simulink model "Control_model_10DOF_fin"  (R2016b)
(part 17 of 18)

JLcom(2,6)=(2*a2*mshank*cos(theta3 + theta4 - theta5 + theta6 + theta7 + theta8) - 2*lshank*mshank*cos(theta6 - theta3 - theta2 + theta7 + theta8) + 2*a2*mshank*cos(theta3 - theta4 + theta5 + theta6 + theta7 + theta8) + 2*a2*mthigh*cos(theta3 + theta4 - theta5 + theta6 + theta7 + theta8) + 2*a2*mthigh*cos(theta3 - theta4 + theta5 + theta6 + theta7 + theta8) - lthigh*mthigh*cos(theta3 + theta4 - theta5 + theta6 + theta7 + theta8) - lthigh*mthigh*cos(theta3 - theta4 + theta5 + theta6 + theta7 + theta8) + 4*a2*mshank*cos(theta6 - theta3 + theta7 + theta8) + 4*a2*mthigh*cos(theta6 - theta3 + theta7 + theta8) - 2*lthigh*mthigh*cos(theta6 - theta3 + theta7 + theta8) - 4*a4*mshank*sin(theta6 - theta5 + theta7 + theta8) - 4*a4*mthigh*sin(theta6 - theta5 + theta7 + theta8) - 4*a4*mtrunk*sin(theta6 - theta5 + theta7 + theta8) - 4*a1*mshank*cos(theta2 + theta3 + theta6 + theta7 + theta8) - 4*mtrunk*ypelvis*cos(theta6 - theta5 + theta7 + theta8) + 2*a1*mshank*cos(theta4 - theta3 - theta2 - theta5 + theta6 + theta7 + theta8) + 2*a1*mshank*cos(theta5 - theta3 - theta4 - theta2 + theta6 + theta7 + theta8) + 2*lshank*mshank*cos(theta2 + theta3 + theta6 + theta7 + theta8) + 4*mtrunk*xpelvis*sin(theta6 - theta5 + theta7 + theta8) - lshank*mshank*cos(theta4 - theta3 - theta2 - theta5 + theta6 + theta7 + theta8) - lshank*mshank*cos(theta5 - theta3 - theta4 - theta2 + theta6 + theta7 + theta8) + 2*a2*mshank*cos(theta4 - theta3 - theta5 + theta6 + theta7 + theta8) + 2*a2*mshank*cos(theta5 - theta4 - theta3 + theta6 + theta7 + theta8) + 2*a2*mthigh*cos(theta4 - theta3 - theta5 + theta6 + theta7 + theta8) + 2*a2*mthigh*cos(theta5 - theta4 - theta3 + theta6 + theta7 + theta8) - lthigh*mthigh*cos(theta4 - theta3 - theta5 + theta6 + theta7 + theta8) - lthigh*mthigh*cos(theta5 - theta4 - theta3 + theta6 + theta7 + theta8) - 8*mtrunk*zpelvis*sin(theta6 + theta7 + theta8) + 2*a1*mshank*cos(theta2 + theta3 + theta4 - theta5 + theta6 + theta7 + theta8) + 2*a1*mshank*cos(theta2 + theta3 - theta4 + theta5 + theta6 + theta7 + theta8) - lshank*mshank*cos(theta2 + theta3 + theta4 - theta5 + theta6 + theta7 + theta8) - lshank*mshank*cos(theta2 + theta3 - theta4 + theta5 + theta6 + theta7 + theta8) + 4*d3*mshank*sin(theta4 - theta5 + theta6 + theta7 + theta8) - 4*d3*mshank*sin(theta5 - theta4 + theta6 + theta7 + theta8) + 4*d3*mthigh*sin(theta4 - theta5 + theta6 + theta7 + theta8) - 4*d3*mthigh*sin(theta5 - theta4 + theta6 + theta7 + theta8) - 4*a2*mshank*cos(theta3 + theta6 + theta7 + theta8) - 4*a2*mthigh*cos(theta3 + theta6 + theta7 + theta8) + 2*lthigh*mthigh*cos(theta3 + theta6 + theta7 + theta8) + 4*a4*mshank*sin(theta5 + theta6 + theta7 + theta8) + 4*a4*mthigh*sin(theta5 + theta6 + theta7 + theta8) + 4*a4*mtrunk*sin(theta5 + theta6 + theta7 + theta8) - 4*mtrunk*ypelvis*cos(theta5 + theta6 + theta7 + theta8) - 4*mtrunk*xpelvis*sin(theta5 + theta6 + theta7 + theta8) + 4*a1*mshank*cos(theta6 - theta3 - theta2 + theta7 + theta8))/(8*(2*mshank + 2*mthigh + mtrunk));
JLcom(2,7)=(2*a2*mshank*cos(theta3 + theta4 - theta5 + theta6 + theta7 + theta8) - 2*lshank*mshank*cos(theta6 - theta3 - theta2 + theta7 + theta8) + 2*a2*mshank*cos(theta3 - theta4 + theta5 + theta6 + theta7 + theta8) + 2*a2*mthigh*cos(theta3 + theta4 - theta5 + theta6 + theta7 + theta8) + 2*a2*mthigh*cos(theta3 - theta4 + theta5 + theta6 + theta7 + theta8) - lthigh*mthigh*cos(theta3 + theta4 - theta5 + theta6 + theta7 + theta8) - lthigh*mthigh*cos(theta3 - theta4 + theta5 + theta6 + theta7 + theta8) + 4*a2*mshank*cos(theta6 - theta3 + theta7 + theta8) + 4*a2*mthigh*cos(theta6 - theta3 + theta7 + theta8) - 2*lthigh*mthigh*cos(theta6 - theta3 + theta7 + theta8) - 4*a4*mshank*sin(theta6 - theta5 + theta7 + theta8) - 4*a4*mthigh*sin(theta6 - theta5 + theta7 + theta8) - 4*a4*mtrunk*sin(theta6 - theta5 + theta7 + theta8) - 4*a1*mshank*cos(theta2 + theta3 + theta6 + theta7 + theta8) - 4*mtrunk*ypelvis*cos(theta6 - theta5 + theta7 + theta8) + 2*a1*mshank*cos(theta4 - theta3 - theta2 - theta5 + theta6 + theta7 + theta8) + 2*a1*mshank*cos(theta5 - theta3 - theta4 - theta2 + theta6 + theta7 + theta8) + 2*lshank*mshank*cos(theta2 + theta3 + theta6 + theta7 + theta8) + 4*mtrunk*xpelvis*sin(theta6 - theta5 + theta7 + theta8) - lshank*mshank*cos(theta4 - theta3 - theta2 - theta5 + theta6 + theta7 + theta8) - lshank*mshank*cos(theta5 - theta3 - theta4 - theta2 + theta6 + theta7 + theta8) + 2*a2*mshank*cos(theta4 - theta3 - theta5 + theta6 + theta7 + theta8) + 2*a2*mshank*cos(theta5 - theta4 - theta3 + theta6 + theta7 + theta8) + 2*a2*mthigh*cos(theta4 - theta3 - theta5 + theta6 + theta7 + theta8) + 2*a2*mthigh*cos(theta5 - theta4 - theta3 + theta6 + theta7 + theta8) - lthigh*mthigh*cos(theta4 - theta3 - theta5 + theta6 + theta7 + theta8) - lthigh*mthigh*cos(theta5 - theta4 - theta3 + theta6 + theta7 + theta8) - 8*mtrunk*zpelvis*sin(theta6 + theta7 + theta8) + 2*a1*mshank*cos(theta2 + theta3 + theta4 - theta5 + theta6 + theta7 + theta8) + 2*a1*mshank*cos(theta2 + theta3 - theta4 + theta5 + theta6 + theta7 + theta8) - lshank*mshank*cos(theta2 + theta3 + theta4 - theta5 + theta6 + theta7 + theta8) - lshank*mshank*cos(theta2 + theta3 - theta4 + theta5 + theta6 + theta7 + theta8) + 4*d3*mshank*sin(theta4 - theta5 + theta6 + theta7 + theta8) - 4*d3*mshank*sin(theta5 - theta4 + theta6 + theta7 + theta8) + 4*d3*mthigh*sin(theta4 - theta5 + theta6 + theta7 + theta8) - 4*d3*mthigh*sin(theta5 - theta4 + theta6 + theta7 + theta8) - 4*a2*mshank*cos(theta3 + theta6 + theta7 + theta8) - 4*a2*mthigh*cos(theta3 + theta6 + theta7 + theta8) + 2*lthigh*mthigh*cos(theta3 + theta6 + theta7 + theta8) + 4*a4*mshank*sin(theta5 + theta6 + theta7 + theta8) + 4*a4*mthigh*sin(theta5 + theta6 + theta7 + theta8) + 4*a4*mtrunk*sin(theta5 + theta6 + theta7 + theta8) + 8*a6*mshank*cos(theta7 + theta8) + 16*a6*mthigh*cos(theta7 + theta8) + 8*a6*mtrunk*cos(theta7 + theta8) - 4*mtrunk*ypelvis*cos(theta5 + theta6 + theta7 + theta8) + 4*lthigh*mthigh*cos(theta7 + theta8) - 4*mtrunk*xpelvis*sin(theta5 + theta6 + theta7 + theta8) + 4*a1*mshank*cos(theta6 - theta3 - theta2 + theta7 + theta8))/(8*(2*mshank + 2*mthigh + mtrunk));
JLcom(2,8)=(16*a7*mshank*cos(theta8) - 2*lshank*mshank*cos(theta6 - theta3 - theta2 + theta7 + theta8) + 16*a7*mthigh*cos(theta8) + 8*a7*mtrunk*cos(theta8) + 2*a2*mshank*cos(theta3 + theta4 - theta5 + theta6 + theta7 + theta8) + 2*a2*mshank*cos(theta3 - theta4 + theta5 + theta6 + theta7 + theta8) + 2*a2*mthigh*cos(theta3 + theta4 - theta5 + theta6 + theta7 + theta8) + 2*a2*mthigh*cos(theta3 - theta4 + theta5 + theta6 + theta7 + theta8) + 4*lshank*mshank*cos(theta8) - lthigh*mthigh*cos(theta3 + theta4 - theta5 + theta6 + theta7 + theta8) - lthigh*mthigh*cos(theta3 - theta4 + theta5 + theta6 + theta7 + theta8) + 4*a2*mshank*cos(theta6 - theta3 + theta7 + theta8) + 4*a2*mthigh*cos(theta6 - theta3 + theta7 + theta8) - 2*lthigh*mthigh*cos(theta6 - theta3 + theta7 + theta8) - 4*a4*mshank*sin(theta6 - theta5 + theta7 + theta8) - 4*a4*mthigh*sin(theta6 - theta5 + theta7 + theta8) - 4*a4*mtrunk*sin(theta6 - theta5 + theta7 + theta8) - 4*a1*mshank*cos(theta2 + theta3 + theta6 + theta7 + theta8) - 4*mtrunk*ypelvis*cos(theta6 - theta5 + theta7 + theta8) + 2*a1*mshank*cos(theta4 - theta3 - theta2 - theta5 + theta6 + theta7 + theta8) + 2*a1*mshank*cos(theta5 - theta3 - theta4 - theta2 + theta6 + theta7 + theta8) + 2*lshank*mshank*cos(theta2 + theta3 + theta6 + theta7 + theta8) + 4*mtrunk*xpelvis*sin(theta6 - theta5 + theta7 + theta8) - lshank*mshank*cos(theta4 - theta3 - theta2 - theta5 + theta6 + theta7 + theta8) - lshank*mshank*cos(theta5 - theta3 - theta4 - theta2 + theta6 + theta7 + theta8) + 2*a2*mshank*cos(theta4 - theta3 - theta5 + theta6 + theta7 + theta8) + 2*a2*mshank*cos(theta5 - theta4 - theta3 + theta6 + theta7 + theta8) + 2*a2*mthigh*cos(theta4 - theta3 - theta5 + theta6 + theta7 + theta8) + 2*a2*mthigh*cos(theta5 - theta4 - theta3 + theta6 + theta7 + theta8) - lthigh*mthigh*cos(theta4 - theta3 - theta5 + theta6 + theta7 + theta8) - lthigh*mthigh*cos(theta5 - theta4 - theta3 + theta6 + theta7 + theta8) - 8*mtrunk*zpelvis*sin(theta6 + theta7 + theta8) + 2*a1*mshank*cos(theta2 + theta3 + theta4 - theta5 + theta6 + theta7 + theta8) + 2*a1*mshank*cos(theta2 + theta3 - theta4 + theta5 + theta6 + theta7 + theta8) - lshank*mshank*cos(theta2 + theta3 + theta4 - theta5 + theta6 + theta7 + theta8) - lshank*mshank*cos(theta2 + theta3 - theta4 + theta5 + theta6 + theta7 + theta8) + 4*d3*mshank*sin(theta4 - theta5 + theta6 + theta7 + theta8) - 4*d3*mshank*sin(theta5 - theta4 + theta6 + theta7 + theta8) + 4*d3*mthigh*sin(theta4 - theta5 + theta6 + theta7 + theta8) - 4*d3*mthigh*sin(theta5 - theta4 + theta6 + theta7 + theta8) - 4*a2*mshank*cos(theta3 + theta6 + theta7 + theta8) - 4*a2*mthigh*cos(theta3 + theta6 + theta7 + theta8) + 2*lthigh*mthigh*cos(theta3 + theta6 + theta7 + theta8) + 4*a4*mshank*sin(theta5 + theta6 + theta7 + theta8) + 4*a4*mthigh*sin(theta5 + theta6 + theta7 + theta8) + 4*a4*mtrunk*sin(theta5 + theta6 + theta7 + theta8) + 8*a6*mshank*cos(theta7 + theta8) + 16*a6*mthigh*cos(theta7 + theta8) + 8*a6*mtrunk*cos(theta7 + theta8) - 4*mtrunk*ypelvis*cos(theta5 + theta6 + theta7 + theta8) + 4*lthigh*mthigh*cos(theta7 + theta8) - 4*mtrunk*xpelvis*sin(theta5 + theta6 + theta7 + theta8) + 4*a1*mshank*cos(theta6 - theta3 - theta2 + theta7 + theta8))/(8*(2*mshank + 2*mthigh + mtrunk));

JLcom(3,5)=(2*a4*mshank*cos(theta9)*sin(theta5) - 2*mtrunk*xpelvis*cos(theta9)*sin(theta5) + 2*a4*mthigh*cos(theta9)*sin(theta5) + 2*a4*mtrunk*cos(theta9)*sin(theta5) - 2*mtrunk*ypelvis*cos(theta5)*cos(theta9) - 2*d3*mshank*cos(theta4)*cos(theta9)*sin(theta5) + 2*d3*mshank*cos(theta5)*cos(theta9)*sin(theta4) - 2*d3*mthigh*cos(theta4)*cos(theta9)*sin(theta5) + 2*d3*mthigh*cos(theta5)*cos(theta9)*sin(theta4) + 2*a2*mshank*cos(theta3)*cos(theta4)*cos(theta5)*cos(theta9) + 2*a2*mthigh*cos(theta3)*cos(theta4)*cos(theta5)*cos(theta9) - lthigh*mthigh*cos(theta3)*cos(theta4)*cos(theta5)*cos(theta9) + 2*a2*mshank*cos(theta3)*cos(theta9)*sin(theta4)*sin(theta5) + 2*a2*mthigh*cos(theta3)*cos(theta9)*sin(theta4)*sin(theta5) - lthigh*mthigh*cos(theta3)*cos(theta9)*sin(theta4)*sin(theta5) + 2*a1*mshank*cos(theta2)*cos(theta3)*cos(theta4)*cos(theta5)*cos(theta9) - lshank*mshank*cos(theta2)*cos(theta3)*cos(theta4)*cos(theta5)*cos(theta9) + 2*a4*mshank*cos(theta5)*cos(theta6)*cos(theta7)*cos(theta8)*sin(theta9) + 2*a4*mthigh*cos(theta5)*cos(theta6)*cos(theta7)*cos(theta8)*sin(theta9) + 2*a4*mtrunk*cos(theta5)*cos(theta6)*cos(theta7)*cos(theta8)*sin(theta9) + 2*a1*mshank*cos(theta2)*cos(theta3)*cos(theta9)*sin(theta4)*sin(theta5) - 2*a1*mshank*cos(theta4)*cos(theta5)*cos(theta9)*sin(theta2)*sin(theta3) - 2*mtrunk*xpelvis*cos(theta5)*cos(theta6)*cos(theta7)*cos(theta8)*sin(theta9) - lshank*mshank*cos(theta2)*cos(theta3)*cos(theta9)*sin(theta4)*sin(theta5) + lshank*mshank*cos(theta4)*cos(theta5)*cos(theta9)*sin(theta2)*sin(theta3) - 2*a4*mshank*cos(theta5)*cos(theta6)*sin(theta7)*sin(theta8)*sin(theta9) - 2*a4*mshank*cos(theta5)*cos(theta7)*sin(theta6)*sin(theta8)*sin(theta9) - 2*a4*mshank*cos(theta5)*cos(theta8)*sin(theta6)*sin(theta7)*sin(theta9) - 2*a4*mthigh*cos(theta5)*cos(theta6)*sin(theta7)*sin(theta8)*sin(theta9) - 2*a4*mthigh*cos(theta5)*cos(theta7)*sin(theta6)*sin(theta8)*sin(theta9) - 2*a4*mthigh*cos(theta5)*cos(theta8)*sin(theta6)*sin(theta7)*sin(theta9) - 2*a4*mtrunk*cos(theta5)*cos(theta6)*sin(theta7)*sin(theta8)*sin(theta9) - 2*a4*mtrunk*cos(theta5)*cos(theta7)*sin(theta6)*sin(theta8)*sin(theta9) - 2*a4*mtrunk*cos(theta5)*cos(theta8)*sin(theta6)*sin(theta7)*sin(theta9) + 2*mtrunk*ypelvis*cos(theta6)*cos(theta7)*cos(theta8)*sin(theta5)*sin(theta9) - 2*a1*mshank*cos(theta9)*sin(theta2)*sin(theta3)*sin(theta4)*sin(theta5) + 2*mtrunk*xpelvis*cos(theta5)*cos(theta6)*sin(theta7)*sin(theta8)*sin(theta9) + 2*mtrunk*xpelvis*cos(theta5)*cos(theta7)*sin(theta6)*sin(theta8)*sin(theta9) + 2*mtrunk*xpelvis*cos(theta5)*cos(theta8)*sin(theta6)*sin(theta7)*sin(theta9) + lshank*mshank*cos(theta9)*sin(theta2)*sin(theta3)*sin(theta4)*sin(theta5) - 2*mtrunk*ypelvis*cos(theta6)*sin(theta5)*sin(theta7)*sin(theta8)*sin(theta9) - 2*mtrunk*ypelvis*cos(theta7)*sin(theta5)*sin(theta6)*sin(theta8)*sin(theta9) - 2*mtrunk*ypelvis*cos(theta8)*sin(theta5)*sin(theta6)*sin(theta7)*sin(theta9) - 2*d3*mshank*cos(theta4)*cos(theta5)*cos(theta6)*cos(theta7)*cos(theta8)*sin(theta9) - 2*d3*mthigh*cos(theta4)*cos(theta5)*cos(theta6)*cos(theta7)*cos(theta8)*sin(theta9) + 2*d3*mshank*cos(theta4)*cos(theta5)*cos(theta6)*sin(theta7)*sin(theta8)*sin(theta9) + 2*d3*mshank*cos(theta4)*cos(theta5)*cos(theta7)*sin(theta6)*sin(theta8)*sin(theta9) + 2*d3*mshank*cos(theta4)*cos(theta5)*cos(theta8)*sin(theta6)*sin(theta7)*sin(theta9) - 2*d3*mshank*cos(theta6)*cos(theta7)*cos(theta8)*sin(theta4)*sin(theta5)*sin(theta9) + 2*d3*mthigh*cos(theta4)*cos(theta5)*cos(theta6)*sin(theta7)*sin(theta8)*sin(theta9) + 2*d3*mthigh*cos(theta4)*cos(theta5)*cos(theta7)*sin(theta6)*sin(theta8)*sin(theta9) + 2*d3*mthigh*cos(theta4)*cos(theta5)*cos(theta8)*sin(theta6)*sin(theta7)*sin(theta9) - 2*d3*mthigh*cos(theta6)*cos(theta7)*cos(theta8)*sin(theta4)*sin(theta5)*sin(theta9) + 2*d3*mshank*cos(theta6)*sin(theta4)*sin(theta5)*sin(theta7)*sin(theta8)*sin(theta9) + 2*d3*mshank*cos(theta7)*sin(theta4)*sin(theta5)*sin(theta6)*sin(theta8)*sin(theta9) + 2*d3*mshank*cos(theta8)*sin(theta4)*sin(theta5)*sin(theta6)*sin(theta7)*sin(theta9) + 2*d3*mthigh*cos(theta6)*sin(theta4)*sin(theta5)*sin(theta7)*sin(theta8)*sin(theta9) + 2*d3*mthigh*cos(theta7)*sin(theta4)*sin(theta5)*sin(theta6)*sin(theta8)*sin(theta9) + 2*d3*mthigh*cos(theta8)*sin(theta4)*sin(theta5)*sin(theta6)*sin(theta7)*sin(theta9) - 2*a2*mshank*cos(theta3)*cos(theta4)*cos(theta6)*cos(theta7)*cos(theta8)*sin(theta5)*sin(theta9) + 2*a2*mshank*cos(theta3)*cos(theta5)*cos(theta6)*cos(theta7)*cos(theta8)*sin(theta4)*sin(theta9) - 2*a2*mthigh*cos(theta3)*cos(theta4)*cos(theta6)*cos(theta7)*cos(theta8)*sin(theta5)*sin(theta9) + 2*a2*mthigh*cos(theta3)*cos(theta5)*cos(theta6)*cos(theta7)*cos(theta8)*sin(theta4)*sin(theta9) + lthigh*mthigh*cos(theta3)*cos(theta4)*cos(theta6)*cos(theta7)*cos(theta8)*sin(theta5)*sin(theta9) - lthigh*mthigh*cos(theta3)*cos(theta5)*cos(theta6)*cos(theta7)*cos(theta8)*sin(theta4)*sin(theta9) + 2*a2*mshank*cos(theta3)*cos(theta4)*cos(theta6)*sin(theta5)*sin(theta7)*sin(theta8)*sin(theta9) + 2*a2*mshank*cos(theta3)*cos(theta4)*cos(theta7)*sin(theta5)*sin(theta6)*sin(theta8)*sin(theta9) + 2*a2*mshank*cos(theta3)*cos(theta4)*cos(theta8)*sin(theta5)*sin(theta6)*sin(theta7)*sin(theta9) - 2*a2*mshank*cos(theta3)*cos(theta5)*cos(theta6)*sin(theta4)*sin(theta7)*sin(theta8)*sin(theta9) - 2*a2*mshank*cos(theta3)*cos(theta5)*cos(theta7)*sin(theta4)*sin(theta6)*sin(theta8)*sin(theta9) - 2*a2*mshank*cos(theta3)*cos(theta5)*cos(theta8)*sin(theta4)*sin(theta6)*sin(theta7)*sin(theta9) + 2*a2*mthigh*cos(theta3)*cos(theta4)*cos(theta6)*sin(theta5)*sin(theta7)*sin(theta8)*sin(theta9) + 2*a2*mthigh*cos(theta3)*cos(theta4)*cos(theta7)*sin(theta5)*sin(theta6)*sin(theta8)*sin(theta9) + 2*a2*mthigh*cos(theta3)*cos(theta4)*cos(theta8)*sin(theta5)*sin(theta6)*sin(theta7)*sin(theta9) - 2*a2*mthigh*cos(theta3)*cos(theta5)*cos(theta6)*sin(theta4)*sin(theta7)*sin(theta8)*sin(theta9) - 2*a2*mthigh*cos(theta3)*cos(theta5)*cos(theta7)*sin(theta4)*sin(theta6)*sin(theta8)*sin(theta9) - 2*a2*mthigh*cos(theta3)*cos(theta5)*cos(theta8)*sin(theta4)*sin(theta6)*sin(theta7)*sin(theta9) - lthigh*mthigh*cos(theta3)*cos(theta4)*cos(theta6)*sin(theta5)*sin(theta7)*sin(theta8)*sin(theta9) - lthigh*mthigh*cos(theta3)*cos(theta4)*cos(theta7)*sin(theta5)*sin(theta6)*sin(theta8)*sin(theta9) - lthigh*mthigh*cos(theta3)*cos(theta4)*cos(theta8)*sin(theta5)*sin(theta6)*sin(theta7)*sin(theta9) + lthigh*mthigh*cos(theta3)*cos(theta5)*cos(theta6)*sin(theta4)*sin(theta7)*sin(theta8)*sin(theta9) + lthigh*mthigh*cos(theta3)*cos(theta5)*cos(theta7)*sin(theta4)*sin(theta6)*sin(theta8)*sin(theta9) + lthigh*mthigh*cos(theta3)*cos(theta5)*cos(theta8)*sin(theta4)*sin(theta6)*sin(theta7)*sin(theta9) - 2*a1*mshank*cos(theta2)*cos(theta3)*cos(theta4)*cos(theta6)*cos(theta7)*cos(theta8)*sin(theta5)*sin(theta9) + 2*a1*mshank*cos(theta2)*cos(theta3)*cos(theta5)*cos(theta6)*cos(theta7)*cos(theta8)*sin(theta4)*sin(theta9) + lshank*mshank*cos(theta2)*cos(theta3)*cos(theta4)*cos(theta6)*cos(theta7)*cos(theta8)*sin(theta5)*sin(theta9) - lshank*mshank*cos(theta2)*cos(theta3)*cos(theta5)*cos(theta6)*cos(theta7)*cos(theta8)*sin(theta4)*sin(theta9) + 2*a1*mshank*cos(theta2)*cos(theta3)*cos(theta4)*cos(theta6)*sin(theta5)*sin(theta7)*sin(theta8)*sin(theta9) + 2*a1*mshank*cos(theta2)*cos(theta3)*cos(theta4)*cos(theta7)*sin(theta5)*sin(theta6)*sin(theta8)*sin(theta9) + 2*a1*mshank*cos(theta2)*cos(theta3)*cos(theta4)*cos(theta8)*sin(theta5)*sin(theta6)*sin(theta7)*sin(theta9) - 2*a1*mshank*cos(theta2)*cos(theta3)*cos(theta5)*cos(theta6)*sin(theta4)*sin(theta7)*sin(theta8)*sin(theta9) - 2*a1*mshank*cos(theta2)*cos(theta3)*cos(theta5)*cos(theta7)*sin(theta4)*sin(theta6)*sin(theta8)*sin(theta9) - 2*a1*mshank*cos(theta2)*cos(theta3)*cos(theta5)*cos(theta8)*sin(theta4)*sin(theta6)*sin(theta7)*sin(theta9) + 2*a1*mshank*cos(theta4)*cos(theta6)*cos(theta7)*cos(theta8)*sin(theta2)*sin(theta3)*sin(theta5)*sin(theta9) - 2*a1*mshank*cos(theta5)*cos(theta6)*cos(theta7)*cos(theta8)*sin(theta2)*sin(theta3)*sin(theta4)*sin(theta9) - lshank*mshank*cos(theta2)*cos(theta3)*cos(theta4)*cos(theta6)*sin(theta5)*sin(theta7)*sin(theta8)*sin(theta9) - lshank*mshank*cos(theta2)*cos(theta3)*cos(theta4)*cos(theta7)*sin(theta5)*sin(theta6)*sin(theta8)*sin(theta9) - lshank*mshank*cos(theta2)*cos(theta3)*cos(theta4)*cos(theta8)*sin(theta5)*sin(theta6)*sin(theta7)*sin(theta9) + lshank*mshank*cos(theta2)*cos(theta3)*cos(theta5)*cos(theta6)*sin(theta4)*sin(theta7)*sin(theta8)*sin(theta9) + lshank*mshank*cos(theta2)*cos(theta3)*cos(theta5)*cos(theta7)*sin(theta4)*sin(theta6)*sin(theta8)*sin(theta9) + lshank*mshank*cos(theta2)*cos(theta3)*cos(theta5)*cos(theta8)*sin(theta4)*sin(theta6)*sin(theta7)*sin(theta9) - lshank*mshank*cos(theta4)*cos(theta6)*cos(theta7)*cos(theta8)*sin(theta2)*sin(theta3)*sin(theta5)*sin(theta9) + lshank*mshank*cos(theta5)*cos(theta6)*cos(theta7)*cos(theta8)*sin(theta2)*sin(theta3)*sin(theta4)*sin(theta9) - 2*a1*mshank*cos(theta4)*cos(theta6)*sin(theta2)*sin(theta3)*sin(theta5)*sin(theta7)*sin(theta8)*sin(theta9) - 2*a1*mshank*cos(theta4)*cos(theta7)*sin(theta2)*sin(theta3)*sin(theta5)*sin(theta6)*sin(theta8)*sin(theta9) - 2*a1*mshank*cos(theta4)*cos(theta8)*sin(theta2)*sin(theta3)*sin(theta5)*sin(theta6)*sin(theta7)*sin(theta9) + 2*a1*mshank*cos(theta5)*cos(theta6)*sin(theta2)*sin(theta3)*sin(theta4)*sin(theta7)*sin(theta8)*sin(theta9) + 2*a1*mshank*cos(theta5)*cos(theta7)*sin(theta2)*sin(theta3)*sin(theta4)*sin(theta6)*sin(theta8)*sin(theta9) + 2*a1*mshank*cos(theta5)*cos(theta8)*sin(theta2)*sin(theta3)*sin(theta4)*sin(theta6)*sin(theta7)*sin(theta9) + lshank*mshank*cos(theta4)*cos(theta6)*sin(theta2)*sin(theta3)*sin(theta5)*sin(theta7)*sin(theta8)*sin(theta9) + lshank*mshank*cos(theta4)*cos(theta7)*sin(theta2)*sin(theta3)*sin(theta5)*sin(theta6)*sin(theta8)*sin(theta9) + lshank*mshank*cos(theta4)*cos(theta8)*sin(theta2)*sin(theta3)*sin(theta5)*sin(theta6)*sin(theta7)*sin(theta9) - lshank*mshank*cos(theta5)*cos(theta6)*sin(theta2)*sin(theta3)*sin(theta4)*sin(theta7)*sin(theta8)*sin(theta9) - lshank*mshank*cos(theta5)*cos(theta7)*sin(theta2)*sin(theta3)*sin(theta4)*sin(theta6)*sin(theta8)*sin(theta9) - lshank*mshank*cos(theta5)*cos(theta8)*sin(theta2)*sin(theta3)*sin(theta4)*sin(theta6)*sin(theta7)*sin(theta9))/(4*mshank + 4*mthigh + 2*mtrunk);
JLcom(3,6)=-(2*mtrunk*zpelvis*cos(theta6)*cos(theta7)*cos(theta8)*sin(theta9) - 2*mtrunk*zpelvis*cos(theta6)*sin(theta7)*sin(theta8)*sin(theta9) - 2*mtrunk*zpelvis*cos(theta7)*sin(theta6)*sin(theta8)*sin(theta9) - 2*mtrunk*zpelvis*cos(theta8)*sin(theta6)*sin(theta7)*sin(theta9) - 2*a2*mshank*cos(theta6)*cos(theta7)*cos(theta8)*sin(theta3)*sin(theta9) - 2*a2*mthigh*cos(theta6)*cos(theta7)*cos(theta8)*sin(theta3)*sin(theta9) + lthigh*mthigh*cos(theta6)*cos(theta7)*cos(theta8)*sin(theta3)*sin(theta9) + 2*a4*mshank*cos(theta6)*cos(theta7)*sin(theta5)*sin(theta8)*sin(theta9) + 2*a4*mshank*cos(theta6)*cos(theta8)*sin(theta5)*sin(theta7)*sin(theta9) + 2*a4*mshank*cos(theta7)*cos(theta8)*sin(theta5)*sin(theta6)*sin(theta9) + 2*a4*mthigh*cos(theta6)*cos(theta7)*sin(theta5)*sin(theta8)*sin(theta9) + 2*a4*mthigh*cos(theta6)*cos(theta8)*sin(theta5)*sin(theta7)*sin(theta9) + 2*a4*mthigh*cos(theta7)*cos(theta8)*sin(theta5)*sin(theta6)*sin(theta9) + 2*a4*mtrunk*cos(theta6)*cos(theta7)*sin(theta5)*sin(theta8)*sin(theta9) + 2*a4*mtrunk*cos(theta6)*cos(theta8)*sin(theta5)*sin(theta7)*sin(theta9) + 2*a4*mtrunk*cos(theta7)*cos(theta8)*sin(theta5)*sin(theta6)*sin(theta9) - 2*mtrunk*ypelvis*cos(theta5)*cos(theta6)*cos(theta7)*sin(theta8)*sin(theta9) - 2*mtrunk*ypelvis*cos(theta5)*cos(theta6)*cos(theta8)*sin(theta7)*sin(theta9) - 2*mtrunk*ypelvis*cos(theta5)*cos(theta7)*cos(theta8)*sin(theta6)*sin(theta9) + 2*a2*mshank*cos(theta6)*sin(theta3)*sin(theta7)*sin(theta8)*sin(theta9) + 2*a2*mshank*cos(theta7)*sin(theta3)*sin(theta6)*sin(theta8)*sin(theta9) + 2*a2*mshank*cos(theta8)*sin(theta3)*sin(theta6)*sin(theta7)*sin(theta9) + 2*a2*mthigh*cos(theta6)*sin(theta3)*sin(theta7)*sin(theta8)*sin(theta9) + 2*a2*mthigh*cos(theta7)*sin(theta3)*sin(theta6)*sin(theta8)*sin(theta9) + 2*a2*mthigh*cos(theta8)*sin(theta3)*sin(theta6)*sin(theta7)*sin(theta9) - 2*mtrunk*xpelvis*cos(theta6)*cos(theta7)*sin(theta5)*sin(theta8)*sin(theta9) - 2*mtrunk*xpelvis*cos(theta6)*cos(theta8)*sin(theta5)*sin(theta7)*sin(theta9) - 2*mtrunk*xpelvis*cos(theta7)*cos(theta8)*sin(theta5)*sin(theta6)*sin(theta9) - lthigh*mthigh*cos(theta6)*sin(theta3)*sin(theta7)*sin(theta8)*sin(theta9) - lthigh*mthigh*cos(theta7)*sin(theta3)*sin(theta6)*sin(theta8)*sin(theta9) - lthigh*mthigh*cos(theta8)*sin(theta3)*sin(theta6)*sin(theta7)*sin(theta9) - 2*a4*mshank*sin(theta5)*sin(theta6)*sin(theta7)*sin(theta8)*sin(theta9) - 2*a4*mthigh*sin(theta5)*sin(theta6)*sin(theta7)*sin(theta8)*sin(theta9) - 2*a4*mtrunk*sin(theta5)*sin(theta6)*sin(theta7)*sin(theta8)*sin(theta9) + 2*mtrunk*ypelvis*cos(theta5)*sin(theta6)*sin(theta7)*sin(theta8)*sin(theta9) + 2*mtrunk*xpelvis*sin(theta5)*sin(theta6)*sin(theta7)*sin(theta8)*sin(theta9) - 2*a1*mshank*cos(theta2)*cos(theta6)*cos(theta7)*cos(theta8)*sin(theta3)*sin(theta9) - 2*a1*mshank*cos(theta3)*cos(theta6)*cos(theta7)*cos(theta8)*sin(theta2)*sin(theta9) + lshank*mshank*cos(theta2)*cos(theta6)*cos(theta7)*cos(theta8)*sin(theta3)*sin(theta9) + lshank*mshank*cos(theta3)*cos(theta6)*cos(theta7)*cos(theta8)*sin(theta2)*sin(theta9) - 2*d3*mshank*cos(theta4)*cos(theta6)*cos(theta7)*sin(theta5)*sin(theta8)*sin(theta9) - 2*d3*mshank*cos(theta4)*cos(theta6)*cos(theta8)*sin(theta5)*sin(theta7)*sin(theta9) - 2*d3*mshank*cos(theta4)*cos(theta7)*cos(theta8)*sin(theta5)*sin(theta6)*sin(theta9) + 2*d3*mshank*cos(theta5)*cos(theta6)*cos(theta7)*sin(theta4)*sin(theta8)*sin(theta9) + 2*d3*mshank*cos(theta5)*cos(theta6)*cos(theta8)*sin(theta4)*sin(theta7)*sin(theta9) + 2*d3*mshank*cos(theta5)*cos(theta7)*cos(theta8)*sin(theta4)*sin(theta6)*sin(theta9) - 2*d3*mthigh*cos(theta4)*cos(theta6)*cos(theta7)*sin(theta5)*sin(theta8)*sin(theta9) - 2*d3*mthigh*cos(theta4)*cos(theta6)*cos(theta8)*sin(theta5)*sin(theta7)*sin(theta9) - 2*d3*mthigh*cos(theta4)*cos(theta7)*cos(theta8)*sin(theta5)*sin(theta6)*sin(theta9) + 2*d3*mthigh*cos(theta5)*cos(theta6)*cos(theta7)*sin(theta4)*sin(theta8)*sin(theta9) + 2*d3*mthigh*cos(theta5)*cos(theta6)*cos(theta8)*sin(theta4)*sin(theta7)*sin(theta9) + 2*d3*mthigh*cos(theta5)*cos(theta7)*cos(theta8)*sin(theta4)*sin(theta6)*sin(theta9) + 2*a1*mshank*cos(theta2)*cos(theta6)*sin(theta3)*sin(theta7)*sin(theta8)*sin(theta9) + 2*a1*mshank*cos(theta2)*cos(theta7)*sin(theta3)*sin(theta6)*sin(theta8)*sin(theta9) + 2*a1*mshank*cos(theta2)*cos(theta8)*sin(theta3)*sin(theta6)*sin(theta7)*sin(theta9) + 2*a1*mshank*cos(theta3)*cos(theta6)*sin(theta2)*sin(theta7)*sin(theta8)*sin(theta9) + 2*a1*mshank*cos(theta3)*cos(theta7)*sin(theta2)*sin(theta6)*sin(theta8)*sin(theta9) + 2*a1*mshank*cos(theta3)*cos(theta8)*sin(theta2)*sin(theta6)*sin(theta7)*sin(theta9) - lshank*mshank*cos(theta2)*cos(theta6)*sin(theta3)*sin(theta7)*sin(theta8)*sin(theta9) - lshank*mshank*cos(theta2)*cos(theta7)*sin(theta3)*sin(theta6)*sin(theta8)*sin(theta9) - lshank*mshank*cos(theta2)*cos(theta8)*sin(theta3)*sin(theta6)*sin(theta7)*sin(theta9) - lshank*mshank*cos(theta3)*cos(theta6)*sin(theta2)*sin(theta7)*sin(theta8)*sin(theta9) - lshank*mshank*cos(theta3)*cos(theta7)*sin(theta2)*sin(theta6)*sin(theta8)*sin(theta9) - lshank*mshank*cos(theta3)*cos(theta8)*sin(theta2)*sin(theta6)*sin(theta7)*sin(theta9) + 2*d3*mshank*cos(theta4)*sin(theta5)*sin(theta6)*sin(theta7)*sin(theta8)*sin(theta9) - 2*d3*mshank*cos(theta5)*sin(theta4)*sin(theta6)*sin(theta7)*sin(theta8)*sin(theta9) + 2*d3*mthigh*cos(theta4)*sin(theta5)*sin(theta6)*sin(theta7)*sin(theta8)*sin(theta9) - 2*d3*mthigh*cos(theta5)*sin(theta4)*sin(theta6)*sin(theta7)*sin(theta8)*sin(theta9) + 2*a2*mshank*cos(theta3)*cos(theta4)*cos(theta5)*cos(theta6)*cos(theta7)*sin(theta8)*sin(theta9) + 2*a2*mshank*cos(theta3)*cos(theta4)*cos(theta5)*cos(theta6)*cos(theta8)*sin(theta7)*sin(theta9) + 2*a2*mshank*cos(theta3)*cos(theta4)*cos(theta5)*cos(theta7)*cos(theta8)*sin(theta6)*sin(theta9) + 2*a2*mthigh*cos(theta3)*cos(theta4)*cos(theta5)*cos(theta6)*cos(theta7)*sin(theta8)*sin(theta9) + 2*a2*mthigh*cos(theta3)*cos(theta4)*cos(theta5)*cos(theta6)*cos(theta8)*sin(theta7)*sin(theta9) + 2*a2*mthigh*cos(theta3)*cos(theta4)*cos(theta5)*cos(theta7)*cos(theta8)*sin(theta6)*sin(theta9) - lthigh*mthigh*cos(theta3)*cos(theta4)*cos(theta5)*cos(theta6)*cos(theta7)*sin(theta8)*sin(theta9) - lthigh*mthigh*cos(theta3)*cos(theta4)*cos(theta5)*cos(theta6)*cos(theta8)*sin(theta7)*sin(theta9) - lthigh*mthigh*cos(theta3)*cos(theta4)*cos(theta5)*cos(theta7)*cos(theta8)*sin(theta6)*sin(theta9) - 2*a2*mshank*cos(theta3)*cos(theta4)*cos(theta5)*sin(theta6)*sin(theta7)*sin(theta8)*sin(theta9) + 2*a2*mshank*cos(theta3)*cos(theta6)*cos(theta7)*sin(theta4)*sin(theta5)*sin(theta8)*sin(theta9) + 2*a2*mshank*cos(theta3)*cos(theta6)*cos(theta8)*sin(theta4)*sin(theta5)*sin(theta7)*sin(theta9) + 2*a2*mshank*cos(theta3)*cos(theta7)*cos(theta8)*sin(theta4)*sin(theta5)*sin(theta6)*sin(theta9) - 2*a2*mthigh*cos(theta3)*cos(theta4)*cos(theta5)*sin(theta6)*sin(theta7)*sin(theta8)*sin(theta9) + 2*a2*mthigh*cos(theta3)*cos(theta6)*cos(theta7)*sin(theta4)*sin(theta5)*sin(theta8)*sin(theta9) + 2*a2*mthigh*cos(theta3)*cos(theta6)*cos(theta8)*sin(theta4)*sin(theta5)*sin(theta7)*sin(theta9) + 2*a2*mthigh*cos(theta3)*cos(theta7)*cos(theta8)*sin(theta4)*sin(theta5)*sin(theta6)*sin(theta9) + lthigh*mthigh*cos(theta3)*cos(theta4)*cos(theta5)*sin(theta6)*sin(theta7)*sin(theta8)*sin(theta9) - lthigh*mthigh*cos(theta3)*cos(theta6)*cos(theta7)*sin(theta4)*sin(theta5)*sin(theta8)*sin(theta9) - lthigh*mthigh*cos(theta3)*cos(theta6)*cos(theta8)*sin(theta4)*sin(theta5)*sin(theta7)*sin(theta9) - lthigh*mthigh*cos(theta3)*cos(theta7)*cos(theta8)*sin(theta4)*sin(theta5)*sin(theta6)*sin(theta9) - 2*a2*mshank*cos(theta3)*sin(theta4)*sin(theta5)*sin(theta6)*sin(theta7)*sin(theta8)*sin(theta9) - 2*a2*mthigh*cos(theta3)*sin(theta4)*sin(theta5)*sin(theta6)*sin(theta7)*sin(theta8)*sin(theta9) + lthigh*mthigh*cos(theta3)*sin(theta4)*sin(theta5)*sin(theta6)*sin(theta7)*sin(theta8)*sin(theta9) + 2*a1*mshank*cos(theta2)*cos(theta3)*cos(theta4)*cos(theta5)*cos(theta6)*cos(theta7)*sin(theta8)*sin(theta9) + 2*a1*mshank*cos(theta2)*cos(theta3)*cos(theta4)*cos(theta5)*cos(theta6)*cos(theta8)*sin(theta7)*sin(theta9) + 2*a1*mshank*cos(theta2)*cos(theta3)*cos(theta4)*cos(theta5)*cos(theta7)*cos(theta8)*sin(theta6)*sin(theta9) - lshank*mshank*cos(theta2)*cos(theta3)*cos(theta4)*cos(theta5)*cos(theta6)*cos(theta7)*sin(theta8)*sin(theta9) - lshank*mshank*cos(theta2)*cos(theta3)*cos(theta4)*cos(theta5)*cos(theta6)*cos(theta8)*sin(theta7)*sin(theta9) - lshank*mshank*cos(theta2)*cos(theta3)*cos(theta4)*cos(theta5)*cos(theta7)*cos(theta8)*sin(theta6)*sin(theta9) - 2*a1*mshank*cos(theta2)*cos(theta3)*cos(theta4)*cos(theta5)*sin(theta6)*sin(theta7)*sin(theta8)*sin(theta9) + 2*a1*mshank*cos(theta2)*cos(theta3)*cos(theta6)*cos(theta7)*sin(theta4)*sin(theta5)*sin(theta8)*sin(theta9) + 2*a1*mshank*cos(theta2)*cos(theta3)*cos(theta6)*cos(theta8)*sin(theta4)*sin(theta5)*sin(theta7)*sin(theta9) + 2*a1*mshank*cos(theta2)*cos(theta3)*cos(theta7)*cos(theta8)*sin(theta4)*sin(theta5)*sin(theta6)*sin(theta9) - 2*a1*mshank*cos(theta4)*cos(theta5)*cos(theta6)*cos(theta7)*sin(theta2)*sin(theta3)*sin(theta8)*sin(theta9) - 2*a1*mshank*cos(theta4)*cos(theta5)*cos(theta6)*cos(theta8)*sin(theta2)*sin(theta3)*sin(theta7)*sin(theta9) - 2*a1*mshank*cos(theta4)*cos(theta5)*cos(theta7)*cos(theta8)*sin(theta2)*sin(theta3)*sin(theta6)*sin(theta9) + lshank*mshank*cos(theta2)*cos(theta3)*cos(theta4)*cos(theta5)*sin(theta6)*sin(theta7)*sin(theta8)*sin(theta9) - lshank*mshank*cos(theta2)*cos(theta3)*cos(theta6)*cos(theta7)*sin(theta4)*sin(theta5)*sin(theta8)*sin(theta9) - lshank*mshank*cos(theta2)*cos(theta3)*cos(theta6)*cos(theta8)*sin(theta4)*sin(theta5)*sin(theta7)*sin(theta9) - lshank*mshank*cos(theta2)*cos(theta3)*cos(theta7)*cos(theta8)*sin(theta4)*sin(theta5)*sin(theta6)*sin(theta9) + lshank*mshank*cos(theta4)*cos(theta5)*cos(theta6)*cos(theta7)*sin(theta2)*sin(theta3)*sin(theta8)*sin(theta9) + lshank*mshank*cos(theta4)*cos(theta5)*cos(theta6)*cos(theta8)*sin(theta2)*sin(theta3)*sin(theta7)*sin(theta9) + lshank*mshank*cos(theta4)*cos(theta5)*cos(theta7)*cos(theta8)*sin(theta2)*sin(theta3)*sin(theta6)*sin(theta9) - 2*a1*mshank*cos(theta2)*cos(theta3)*sin(theta4)*sin(theta5)*sin(theta6)*sin(theta7)*sin(theta8)*sin(theta9) + 2*a1*mshank*cos(theta4)*cos(theta5)*sin(theta2)*sin(theta3)*sin(theta6)*sin(theta7)*sin(theta8)*sin(theta9) - 2*a1*mshank*cos(theta6)*cos(theta7)*sin(theta2)*sin(theta3)*sin(theta4)*sin(theta5)*sin(theta8)*sin(theta9) - 2*a1*mshank*cos(theta6)*cos(theta8)*sin(theta2)*sin(theta3)*sin(theta4)*sin(theta5)*sin(theta7)*sin(theta9) - 2*a1*mshank*cos(theta7)*cos(theta8)*sin(theta2)*sin(theta3)*sin(theta4)*sin(theta5)*sin(theta6)*sin(theta9) + lshank*mshank*cos(theta2)*cos(theta3)*sin(theta4)*sin(theta5)*sin(theta6)*sin(theta7)*sin(theta8)*sin(theta9) - lshank*mshank*cos(theta4)*cos(theta5)*sin(theta2)*sin(theta3)*sin(theta6)*sin(theta7)*sin(theta8)*sin(theta9) + lshank*mshank*cos(theta6)*cos(theta7)*sin(theta2)*sin(theta3)*sin(theta4)*sin(theta5)*sin(theta8)*sin(theta9) + lshank*mshank*cos(theta6)*cos(theta8)*sin(theta2)*sin(theta3)*sin(theta4)*sin(theta5)*sin(theta7)*sin(theta9) + lshank*mshank*cos(theta7)*cos(theta8)*sin(theta2)*sin(theta3)*sin(theta4)*sin(theta5)*sin(theta6)*sin(theta9) + 2*a1*mshank*sin(theta2)*sin(theta3)*sin(theta4)*sin(theta5)*sin(theta6)*sin(theta7)*sin(theta8)*sin(theta9) - lshank*mshank*sin(theta2)*sin(theta3)*sin(theta4)*sin(theta5)*sin(theta6)*sin(theta7)*sin(theta8)*sin(theta9))/(4*mshank + 4*mthigh + 2*mtrunk);
JLcom(3,7)=-(2*a6*mshank*cos(theta7)*sin(theta8)*sin(theta9) + 2*a6*mshank*cos(theta8)*sin(theta7)*sin(theta9) + 4*a6*mthigh*cos(theta7)*sin(theta8)*sin(theta9) + 4*a6*mthigh*cos(theta8)*sin(theta7)*sin(theta9) + 2*a6*mtrunk*cos(theta7)*sin(theta8)*sin(theta9) + 2*a6*mtrunk*cos(theta8)*sin(theta7)*sin(theta9) + lthigh*mthigh*cos(theta7)*sin(theta8)*sin(theta9) + lthigh*mthigh*cos(theta8)*sin(theta7)*sin(theta9) + 2*mtrunk*zpelvis*cos(theta6)*cos(theta7)*cos(theta8)*sin(theta9) - 2*mtrunk*zpelvis*cos(theta6)*sin(theta7)*sin(theta8)*sin(theta9) - 2*mtrunk*zpelvis*cos(theta7)*sin(theta6)*sin(theta8)*sin(theta9) - 2*mtrunk*zpelvis*cos(theta8)*sin(theta6)*sin(theta7)*sin(theta9) - 2*a2*mshank*cos(theta6)*cos(theta7)*cos(theta8)*sin(theta3)*sin(theta9) - 2*a2*mthigh*cos(theta6)*cos(theta7)*cos(theta8)*sin(theta3)*sin(theta9) + lthigh*mthigh*cos(theta6)*cos(theta7)*cos(theta8)*sin(theta3)*sin(theta9) + 2*a4*mshank*cos(theta6)*cos(theta7)*sin(theta5)*sin(theta8)*sin(theta9) + 2*a4*mshank*cos(theta6)*cos(theta8)*sin(theta5)*sin(theta7)*sin(theta9) + 2*a4*mshank*cos(theta7)*cos(theta8)*sin(theta5)*sin(theta6)*sin(theta9) + 2*a4*mthigh*cos(theta6)*cos(theta7)*sin(theta5)*sin(theta8)*sin(theta9) + 2*a4*mthigh*cos(theta6)*cos(theta8)*sin(theta5)*sin(theta7)*sin(theta9) + 2*a4*mthigh*cos(theta7)*cos(theta8)*sin(theta5)*sin(theta6)*sin(theta9) + 2*a4*mtrunk*cos(theta6)*cos(theta7)*sin(theta5)*sin(theta8)*sin(theta9) + 2*a4*mtrunk*cos(theta6)*cos(theta8)*sin(theta5)*sin(theta7)*sin(theta9) + 2*a4*mtrunk*cos(theta7)*cos(theta8)*sin(theta5)*sin(theta6)*sin(theta9) - 2*mtrunk*ypelvis*cos(theta5)*cos(theta6)*cos(theta7)*sin(theta8)*sin(theta9) - 2*mtrunk*ypelvis*cos(theta5)*cos(theta6)*cos(theta8)*sin(theta7)*sin(theta9) - 2*mtrunk*ypelvis*cos(theta5)*cos(theta7)*cos(theta8)*sin(theta6)*sin(theta9) + 2*a2*mshank*cos(theta6)*sin(theta3)*sin(theta7)*sin(theta8)*sin(theta9) + 2*a2*mshank*cos(theta7)*sin(theta3)*sin(theta6)*sin(theta8)*sin(theta9) + 2*a2*mshank*cos(theta8)*sin(theta3)*sin(theta6)*sin(theta7)*sin(theta9) + 2*a2*mthigh*cos(theta6)*sin(theta3)*sin(theta7)*sin(theta8)*sin(theta9) + 2*a2*mthigh*cos(theta7)*sin(theta3)*sin(theta6)*sin(theta8)*sin(theta9) + 2*a2*mthigh*cos(theta8)*sin(theta3)*sin(theta6)*sin(theta7)*sin(theta9) - 2*mtrunk*xpelvis*cos(theta6)*cos(theta7)*sin(theta5)*sin(theta8)*sin(theta9) - 2*mtrunk*xpelvis*cos(theta6)*cos(theta8)*sin(theta5)*sin(theta7)*sin(theta9) - 2*mtrunk*xpelvis*cos(theta7)*cos(theta8)*sin(theta5)*sin(theta6)*sin(theta9) - lthigh*mthigh*cos(theta6)*sin(theta3)*sin(theta7)*sin(theta8)*sin(theta9) - lthigh*mthigh*cos(theta7)*sin(theta3)*sin(theta6)*sin(theta8)*sin(theta9) - lthigh*mthigh*cos(theta8)*sin(theta3)*sin(theta6)*sin(theta7)*sin(theta9) - 2*a4*mshank*sin(theta5)*sin(theta6)*sin(theta7)*sin(theta8)*sin(theta9) - 2*a4*mthigh*sin(theta5)*sin(theta6)*sin(theta7)*sin(theta8)*sin(theta9) - 2*a4*mtrunk*sin(theta5)*sin(theta6)*sin(theta7)*sin(theta8)*sin(theta9) + 2*mtrunk*ypelvis*cos(theta5)*sin(theta6)*sin(theta7)*sin(theta8)*sin(theta9) + 2*mtrunk*xpelvis*sin(theta5)*sin(theta6)*sin(theta7)*sin(theta8)*sin(theta9) - 2*a1*mshank*cos(theta2)*cos(theta6)*cos(theta7)*cos(theta8)*sin(theta3)*sin(theta9) - 2*a1*mshank*cos(theta3)*cos(theta6)*cos(theta7)*cos(theta8)*sin(theta2)*sin(theta9) + lshank*mshank*cos(theta2)*cos(theta6)*cos(theta7)*cos(theta8)*sin(theta3)*sin(theta9) + lshank*mshank*cos(theta3)*cos(theta6)*cos(theta7)*cos(theta8)*sin(theta2)*sin(theta9) - 2*d3*mshank*cos(theta4)*cos(theta6)*cos(theta7)*sin(theta5)*sin(theta8)*sin(theta9) - 2*d3*mshank*cos(theta4)*cos(theta6)*cos(theta8)*sin(theta5)*sin(theta7)*sin(theta9) - 2*d3*mshank*cos(theta4)*cos(theta7)*cos(theta8)*sin(theta5)*sin(theta6)*sin(theta9) + 2*d3*mshank*cos(theta5)*cos(theta6)*cos(theta7)*sin(theta4)*sin(theta8)*sin(theta9) + 2*d3*mshank*cos(theta5)*cos(theta6)*cos(theta8)*sin(theta4)*sin(theta7)*sin(theta9) + 2*d3*mshank*cos(theta5)*cos(theta7)*cos(theta8)*sin(theta4)*sin(theta6)*sin(theta9) - 2*d3*mthigh*cos(theta4)*cos(theta6)*cos(theta7)*sin(theta5)*sin(theta8)*sin(theta9) - 2*d3*mthigh*cos(theta4)*cos(theta6)*cos(theta8)*sin(theta5)*sin(theta7)*sin(theta9) - 2*d3*mthigh*cos(theta4)*cos(theta7)*cos(theta8)*sin(theta5)*sin(theta6)*sin(theta9) + 2*d3*mthigh*cos(theta5)*cos(theta6)*cos(theta7)*sin(theta4)*sin(theta8)*sin(theta9) + 2*d3*mthigh*cos(theta5)*cos(theta6)*cos(theta8)*sin(theta4)*sin(theta7)*sin(theta9) + 2*d3*mthigh*cos(theta5)*cos(theta7)*cos(theta8)*sin(theta4)*sin(theta6)*sin(theta9) + 2*a1*mshank*cos(theta2)*cos(theta6)*sin(theta3)*sin(theta7)*sin(theta8)*sin(theta9) + 2*a1*mshank*cos(theta2)*cos(theta7)*sin(theta3)*sin(theta6)*sin(theta8)*sin(theta9) + 2*a1*mshank*cos(theta2)*cos(theta8)*sin(theta3)*sin(theta6)*sin(theta7)*sin(theta9) + 2*a1*mshank*cos(theta3)*cos(theta6)*sin(theta2)*sin(theta7)*sin(theta8)*sin(theta9) + 2*a1*mshank*cos(theta3)*cos(theta7)*sin(theta2)*sin(theta6)*sin(theta8)*sin(theta9) + 2*a1*mshank*cos(theta3)*cos(theta8)*sin(theta2)*sin(theta6)*sin(theta7)*sin(theta9) - lshank*mshank*cos(theta2)*cos(theta6)*sin(theta3)*sin(theta7)*sin(theta8)*sin(theta9) - lshank*mshank*cos(theta2)*cos(theta7)*sin(theta3)*sin(theta6)*sin(theta8)*sin(theta9) - lshank*mshank*cos(theta2)*cos(theta8)*sin(theta3)*sin(theta6)*sin(theta7)*sin(theta9) - lshank*mshank*cos(theta3)*cos(theta6)*sin(theta2)*sin(theta7)*sin(theta8)*sin(theta9) - lshank*mshank*cos(theta3)*cos(theta7)*sin(theta2)*sin(theta6)*sin(theta8)*sin(theta9) - lshank*mshank*cos(theta3)*cos(theta8)*sin(theta2)*sin(theta6)*sin(theta7)*sin(theta9) + 2*d3*mshank*cos(theta4)*sin(theta5)*sin(theta6)*sin(theta7)*sin(theta8)*sin(theta9) - 2*d3*mshank*cos(theta5)*sin(theta4)*sin(theta6)*sin(theta7)*sin(theta8)*sin(theta9) + 2*d3*mthigh*cos(theta4)*sin(theta5)*sin(theta6)*sin(theta7)*sin(theta8)*sin(theta9) - 2*d3*mthigh*cos(theta5)*sin(theta4)*sin(theta6)*sin(theta7)*sin(theta8)*sin(theta9) + 2*a2*mshank*cos(theta3)*cos(theta4)*cos(theta5)*cos(theta6)*cos(theta7)*sin(theta8)*sin(theta9) + 2*a2*mshank*cos(theta3)*cos(theta4)*cos(theta5)*cos(theta6)*cos(theta8)*sin(theta7)*sin(theta9) + 2*a2*mshank*cos(theta3)*cos(theta4)*cos(theta5)*cos(theta7)*cos(theta8)*sin(theta6)*sin(theta9) + 2*a2*mthigh*cos(theta3)*cos(theta4)*cos(theta5)*cos(theta6)*cos(theta7)*sin(theta8)*sin(theta9) + 2*a2*mthigh*cos(theta3)*cos(theta4)*cos(theta5)*cos(theta6)*cos(theta8)*sin(theta7)*sin(theta9) + 2*a2*mthigh*cos(theta3)*cos(theta4)*cos(theta5)*cos(theta7)*cos(theta8)*sin(theta6)*sin(theta9) - lthigh*mthigh*cos(theta3)*cos(theta4)*cos(theta5)*cos(theta6)*cos(theta7)*sin(theta8)*sin(theta9) - lthigh*mthigh*cos(theta3)*cos(theta4)*cos(theta5)*cos(theta6)*cos(theta8)*sin(theta7)*sin(theta9) - lthigh*mthigh*cos(theta3)*cos(theta4)*cos(theta5)*cos(theta7)*cos(theta8)*sin(theta6)*sin(theta9) - 2*a2*mshank*cos(theta3)*cos(theta4)*cos(theta5)*sin(theta6)*sin(theta7)*sin(theta8)*sin(theta9) + 2*a2*mshank*cos(theta3)*cos(theta6)*cos(theta7)*sin(theta4)*sin(theta5)*sin(theta8)*sin(theta9) + 2*a2*mshank*cos(theta3)*cos(theta6)*cos(theta8)*sin(theta4)*sin(theta5)*sin(theta7)*sin(theta9) + 2*a2*mshank*cos(theta3)*cos(theta7)*cos(theta8)*sin(theta4)*sin(theta5)*sin(theta6)*sin(theta9) - 2*a2*mthigh*cos(theta3)*cos(theta4)*cos(theta5)*sin(theta6)*sin(theta7)*sin(theta8)*sin(theta9) + 2*a2*mthigh*cos(theta3)*cos(theta6)*cos(theta7)*sin(theta4)*sin(theta5)*sin(theta8)*sin(theta9) + 2*a2*mthigh*cos(theta3)*cos(theta6)*cos(theta8)*sin(theta4)*sin(theta5)*sin(theta7)*sin(theta9) + 2*a2*mthigh*cos(theta3)*cos(theta7)*cos(theta8)*sin(theta4)*sin(theta5)*sin(theta6)*sin(theta9) + lthigh*mthigh*cos(theta3)*cos(theta4)*cos(theta5)*sin(theta6)*sin(theta7)*sin(theta8)*sin(theta9) - lthigh*mthigh*cos(theta3)*cos(theta6)*cos(theta7)*sin(theta4)*sin(theta5)*sin(theta8)*sin(theta9) - lthigh*mthigh*cos(theta3)*cos(theta6)*cos(theta8)*sin(theta4)*sin(theta5)*sin(theta7)*sin(theta9) - lthigh*mthigh*cos(theta3)*cos(theta7)*cos(theta8)*sin(theta4)*sin(theta5)*sin(theta6)*sin(theta9) - 2*a2*mshank*cos(theta3)*sin(theta4)*sin(theta5)*sin(theta6)*sin(theta7)*sin(theta8)*sin(theta9) - 2*a2*mthigh*cos(theta3)*sin(theta4)*sin(theta5)*sin(theta6)*sin(theta7)*sin(theta8)*sin(theta9) + lthigh*mthigh*cos(theta3)*sin(theta4)*sin(theta5)*sin(theta6)*sin(theta7)*sin(theta8)*sin(theta9) + 2*a1*mshank*cos(theta2)*cos(theta3)*cos(theta4)*cos(theta5)*cos(theta6)*cos(theta7)*sin(theta8)*sin(theta9) + 2*a1*mshank*cos(theta2)*cos(theta3)*cos(theta4)*cos(theta5)*cos(theta6)*cos(theta8)*sin(theta7)*sin(theta9) + 2*a1*mshank*cos(theta2)*cos(theta3)*cos(theta4)*cos(theta5)*cos(theta7)*cos(theta8)*sin(theta6)*sin(theta9) - lshank*mshank*cos(theta2)*cos(theta3)*cos(theta4)*cos(theta5)*cos(theta6)*cos(theta7)*sin(theta8)*sin(theta9) - lshank*mshank*cos(theta2)*cos(theta3)*cos(theta4)*cos(theta5)*cos(theta6)*cos(theta8)*sin(theta7)*sin(theta9) - lshank*mshank*cos(theta2)*cos(theta3)*cos(theta4)*cos(theta5)*cos(theta7)*cos(theta8)*sin(theta6)*sin(theta9) - 2*a1*mshank*cos(theta2)*cos(theta3)*cos(theta4)*cos(theta5)*sin(theta6)*sin(theta7)*sin(theta8)*sin(theta9) + 2*a1*mshank*cos(theta2)*cos(theta3)*cos(theta6)*cos(theta7)*sin(theta4)*sin(theta5)*sin(theta8)*sin(theta9) + 2*a1*mshank*cos(theta2)*cos(theta3)*cos(theta6)*cos(theta8)*sin(theta4)*sin(theta5)*sin(theta7)*sin(theta9) + 2*a1*mshank*cos(theta2)*cos(theta3)*cos(theta7)*cos(theta8)*sin(theta4)*sin(theta5)*sin(theta6)*sin(theta9) - 2*a1*mshank*cos(theta4)*cos(theta5)*cos(theta6)*cos(theta7)*sin(theta2)*sin(theta3)*sin(theta8)*sin(theta9) - 2*a1*mshank*cos(theta4)*cos(theta5)*cos(theta6)*cos(theta8)*sin(theta2)*sin(theta3)*sin(theta7)*sin(theta9) - 2*a1*mshank*cos(theta4)*cos(theta5)*cos(theta7)*cos(theta8)*sin(theta2)*sin(theta3)*sin(theta6)*sin(theta9) + lshank*mshank*cos(theta2)*cos(theta3)*cos(theta4)*cos(theta5)*sin(theta6)*sin(theta7)*sin(theta8)*sin(theta9) - lshank*mshank*cos(theta2)*cos(theta3)*cos(theta6)*cos(theta7)*sin(theta4)*sin(theta5)*sin(theta8)*sin(theta9) - lshank*mshank*cos(theta2)*cos(theta3)*cos(theta6)*cos(theta8)*sin(theta4)*sin(theta5)*sin(theta7)*sin(theta9) - lshank*mshank*cos(theta2)*cos(theta3)*cos(theta7)*cos(theta8)*sin(theta4)*sin(theta5)*sin(theta6)*sin(theta9) + lshank*mshank*cos(theta4)*cos(theta5)*cos(theta6)*cos(theta7)*sin(theta2)*sin(theta3)*sin(theta8)*sin(theta9) + lshank*mshank*cos(theta4)*cos(theta5)*cos(theta6)*cos(theta8)*sin(theta2)*sin(theta3)*sin(theta7)*sin(theta9) + lshank*mshank*cos(theta4)*cos(theta5)*cos(theta7)*cos(theta8)*sin(theta2)*sin(theta3)*sin(theta6)*sin(theta9) - 2*a1*mshank*cos(theta2)*cos(theta3)*sin(theta4)*sin(theta5)*sin(theta6)*sin(theta7)*sin(theta8)*sin(theta9) + 2*a1*mshank*cos(theta4)*cos(theta5)*sin(theta2)*sin(theta3)*sin(theta6)*sin(theta7)*sin(theta8)*sin(theta9) - 2*a1*mshank*cos(theta6)*cos(theta7)*sin(theta2)*sin(theta3)*sin(theta4)*sin(theta5)*sin(theta8)*sin(theta9) - 2*a1*mshank*cos(theta6)*cos(theta8)*sin(theta2)*sin(theta3)*sin(theta4)*sin(theta5)*sin(theta7)*sin(theta9) - 2*a1*mshank*cos(theta7)*cos(theta8)*sin(theta2)*sin(theta3)*sin(theta4)*sin(theta5)*sin(theta6)*sin(theta9) + lshank*mshank*cos(theta2)*cos(theta3)*sin(theta4)*sin(theta5)*sin(theta6)*sin(theta7)*sin(theta8)*sin(theta9) - lshank*mshank*cos(theta4)*cos(theta5)*sin(theta2)*sin(theta3)*sin(theta6)*sin(theta7)*sin(theta8)*sin(theta9) + lshank*mshank*cos(theta6)*cos(theta7)*sin(theta2)*sin(theta3)*sin(theta4)*sin(theta5)*sin(theta8)*sin(theta9) + lshank*mshank*cos(theta6)*cos(theta8)*sin(theta2)*sin(theta3)*sin(theta4)*sin(theta5)*sin(theta7)*sin(theta9) + lshank*mshank*cos(theta7)*cos(theta8)*sin(theta2)*sin(theta3)*sin(theta4)*sin(theta5)*sin(theta6)*sin(theta9) + 2*a1*mshank*sin(theta2)*sin(theta3)*sin(theta4)*sin(theta5)*sin(theta6)*sin(theta7)*sin(theta8)*sin(theta9) - lshank*mshank*sin(theta2)*sin(theta3)*sin(theta4)*sin(theta5)*sin(theta6)*sin(theta7)*sin(theta8)*sin(theta9))/(4*mshank + 4*mthigh + 2*mtrunk);
JLcom(3,8)=-(lshank*mshank*sin(theta8)*sin(theta9) + 4*a7*mshank*sin(theta8)*sin(theta9) + 4*a7*mthigh*sin(theta8)*sin(theta9) + 2*a7*mtrunk*sin(theta8)*sin(theta9) + 2*a6*mshank*cos(theta7)*sin(theta8)*sin(theta9) + 2*a6*mshank*cos(theta8)*sin(theta7)*sin(theta9) + 4*a6*mthigh*cos(theta7)*sin(theta8)*sin(theta9) + 4*a6*mthigh*cos(theta8)*sin(theta7)*sin(theta9) + 2*a6*mtrunk*cos(theta7)*sin(theta8)*sin(theta9) + 2*a6*mtrunk*cos(theta8)*sin(theta7)*sin(theta9) + lthigh*mthigh*cos(theta7)*sin(theta8)*sin(theta9) + lthigh*mthigh*cos(theta8)*sin(theta7)*sin(theta9) + 2*mtrunk*zpelvis*cos(theta6)*cos(theta7)*cos(theta8)*sin(theta9) - 2*mtrunk*zpelvis*cos(theta6)*sin(theta7)*sin(theta8)*sin(theta9) - 2*mtrunk*zpelvis*cos(theta7)*sin(theta6)*sin(theta8)*sin(theta9) - 2*mtrunk*zpelvis*cos(theta8)*sin(theta6)*sin(theta7)*sin(theta9) - 2*a2*mshank*cos(theta6)*cos(theta7)*cos(theta8)*sin(theta3)*sin(theta9) - 2*a2*mthigh*cos(theta6)*cos(theta7)*cos(theta8)*sin(theta3)*sin(theta9) + lthigh*mthigh*cos(theta6)*cos(theta7)*cos(theta8)*sin(theta3)*sin(theta9) + 2*a4*mshank*cos(theta6)*cos(theta7)*sin(theta5)*sin(theta8)*sin(theta9) + 2*a4*mshank*cos(theta6)*cos(theta8)*sin(theta5)*sin(theta7)*sin(theta9) + 2*a4*mshank*cos(theta7)*cos(theta8)*sin(theta5)*sin(theta6)*sin(theta9) + 2*a4*mthigh*cos(theta6)*cos(theta7)*sin(theta5)*sin(theta8)*sin(theta9) + 2*a4*mthigh*cos(theta6)*cos(theta8)*sin(theta5)*sin(theta7)*sin(theta9) + 2*a4*mthigh*cos(theta7)*cos(theta8)*sin(theta5)*sin(theta6)*sin(theta9) + 2*a4*mtrunk*cos(theta6)*cos(theta7)*sin(theta5)*sin(theta8)*sin(theta9) + 2*a4*mtrunk*cos(theta6)*cos(theta8)*sin(theta5)*sin(theta7)*sin(theta9) + 2*a4*mtrunk*cos(theta7)*cos(theta8)*sin(theta5)*sin(theta6)*sin(theta9) - 2*mtrunk*ypelvis*cos(theta5)*cos(theta6)*cos(theta7)*sin(theta8)*sin(theta9) - 2*mtrunk*ypelvis*cos(theta5)*cos(theta6)*cos(theta8)*sin(theta7)*sin(theta9) - 2*mtrunk*ypelvis*cos(theta5)*cos(theta7)*cos(theta8)*sin(theta6)*sin(theta9) + 2*a2*mshank*cos(theta6)*sin(theta3)*sin(theta7)*sin(theta8)*sin(theta9) + 2*a2*mshank*cos(theta7)*sin(theta3)*sin(theta6)*sin(theta8)*sin(theta9) + 2*a2*mshank*cos(theta8)*sin(theta3)*sin(theta6)*sin(theta7)*sin(theta9) + 2*a2*mthigh*cos(theta6)*sin(theta3)*sin(theta7)*sin(theta8)*sin(theta9) + 2*a2*mthigh*cos(theta7)*sin(theta3)*sin(theta6)*sin(theta8)*sin(theta9) + 2*a2*mthigh*cos(theta8)*sin(theta3)*sin(theta6)*sin(theta7)*sin(theta9) - 2*mtrunk*xpelvis*cos(theta6)*cos(theta7)*sin(theta5)*sin(theta8)*sin(theta9) - 2*mtrunk*xpelvis*cos(theta6)*cos(theta8)*sin(theta5)*sin(theta7)*sin(theta9) - 2*mtrunk*xpelvis*cos(theta7)*cos(theta8)*sin(theta5)*sin(theta6)*sin(theta9) - lthigh*mthigh*cos(theta6)*sin(theta3)*sin(theta7)*sin(theta8)*sin(theta9) - lthigh*mthigh*cos(theta7)*sin(theta3)*sin(theta6)*sin(theta8)*sin(theta9) - lthigh*mthigh*cos(theta8)*sin(theta3)*sin(theta6)*sin(theta7)*sin(theta9) - 2*a4*mshank*sin(theta5)*sin(theta6)*sin(theta7)*sin(theta8)*sin(theta9) - 2*a4*mthigh*sin(theta5)*sin(theta6)*sin(theta7)*sin(theta8)*sin(theta9) - 2*a4*mtrunk*sin(theta5)*sin(theta6)*sin(theta7)*sin(theta8)*sin(theta9) + 2*mtrunk*ypelvis*cos(theta5)*sin(theta6)*sin(theta7)*sin(theta8)*sin(theta9) + 2*mtrunk*xpelvis*sin(theta5)*sin(theta6)*sin(theta7)*sin(theta8)*sin(theta9) - 2*a1*mshank*cos(theta2)*cos(theta6)*cos(theta7)*cos(theta8)*sin(theta3)*sin(theta9) - 2*a1*mshank*cos(theta3)*cos(theta6)*cos(theta7)*cos(theta8)*sin(theta2)*sin(theta9) + lshank*mshank*cos(theta2)*cos(theta6)*cos(theta7)*cos(theta8)*sin(theta3)*sin(theta9) + lshank*mshank*cos(theta3)*cos(theta6)*cos(theta7)*cos(theta8)*sin(theta2)*sin(theta9) - 2*d3*mshank*cos(theta4)*cos(theta6)*cos(theta7)*sin(theta5)*sin(theta8)*sin(theta9) - 2*d3*mshank*cos(theta4)*cos(theta6)*cos(theta8)*sin(theta5)*sin(theta7)*sin(theta9) - 2*d3*mshank*cos(theta4)*cos(theta7)*cos(theta8)*sin(theta5)*sin(theta6)*sin(theta9) + 2*d3*mshank*cos(theta5)*cos(theta6)*cos(theta7)*sin(theta4)*sin(theta8)*sin(theta9) + 2*d3*mshank*cos(theta5)*cos(theta6)*cos(theta8)*sin(theta4)*sin(theta7)*sin(theta9) + 2*d3*mshank*cos(theta5)*cos(theta7)*cos(theta8)*sin(theta4)*sin(theta6)*sin(theta9) - 2*d3*mthigh*cos(theta4)*cos(theta6)*cos(theta7)*sin(theta5)*sin(theta8)*sin(theta9) - 2*d3*mthigh*cos(theta4)*cos(theta6)*cos(theta8)*sin(theta5)*sin(theta7)*sin(theta9) - 2*d3*mthigh*cos(theta4)*cos(theta7)*cos(theta8)*sin(theta5)*sin(theta6)*sin(theta9) + 2*d3*mthigh*cos(theta5)*cos(theta6)*cos(theta7)*sin(theta4)*sin(theta8)*sin(theta9) + 2*d3*mthigh*cos(theta5)*cos(theta6)*cos(theta8)*sin(theta4)*sin(theta7)*sin(theta9) + 2*d3*mthigh*cos(theta5)*cos(theta7)*cos(theta8)*sin(theta4)*sin(theta6)*sin(theta9) + 2*a1*mshank*cos(theta2)*cos(theta6)*sin(theta3)*sin(theta7)*sin(theta8)*sin(theta9) + 2*a1*mshank*cos(theta2)*cos(theta7)*sin(theta3)*sin(theta6)*sin(theta8)*sin(theta9) + 2*a1*mshank*cos(theta2)*cos(theta8)*sin(theta3)*sin(theta6)*sin(theta7)*sin(theta9) + 2*a1*mshank*cos(theta3)*cos(theta6)*sin(theta2)*sin(theta7)*sin(theta8)*sin(theta9) + 2*a1*mshank*cos(theta3)*cos(theta7)*sin(theta2)*sin(theta6)*sin(theta8)*sin(theta9) + 2*a1*mshank*cos(theta3)*cos(theta8)*sin(theta2)*sin(theta6)*sin(theta7)*sin(theta9) - lshank*mshank*cos(theta2)*cos(theta6)*sin(theta3)*sin(theta7)*sin(theta8)*sin(theta9) - lshank*mshank*cos(theta2)*cos(theta7)*sin(theta3)*sin(theta6)*sin(theta8)*sin(theta9) - lshank*mshank*cos(theta2)*cos(theta8)*sin(theta3)*sin(theta6)*sin(theta7)*sin(theta9) - lshank*mshank*cos(theta3)*cos(theta6)*sin(theta2)*sin(theta7)*sin(theta8)*sin(theta9) - lshank*mshank*cos(theta3)*cos(theta7)*sin(theta2)*sin(theta6)*sin(theta8)*sin(theta9) - lshank*mshank*cos(theta3)*cos(theta8)*sin(theta2)*sin(theta6)*sin(theta7)*sin(theta9) + 2*d3*mshank*cos(theta4)*sin(theta5)*sin(theta6)*sin(theta7)*sin(theta8)*sin(theta9) - 2*d3*mshank*cos(theta5)*sin(theta4)*sin(theta6)*sin(theta7)*sin(theta8)*sin(theta9) + 2*d3*mthigh*cos(theta4)*sin(theta5)*sin(theta6)*sin(theta7)*sin(theta8)*sin(theta9) - 2*d3*mthigh*cos(theta5)*sin(theta4)*sin(theta6)*sin(theta7)*sin(theta8)*sin(theta9) + 2*a2*mshank*cos(theta3)*cos(theta4)*cos(theta5)*cos(theta6)*cos(theta7)*sin(theta8)*sin(theta9) + 2*a2*mshank*cos(theta3)*cos(theta4)*cos(theta5)*cos(theta6)*cos(theta8)*sin(theta7)*sin(theta9) + 2*a2*mshank*cos(theta3)*cos(theta4)*cos(theta5)*cos(theta7)*cos(theta8)*sin(theta6)*sin(theta9) + 2*a2*mthigh*cos(theta3)*cos(theta4)*cos(theta5)*cos(theta6)*cos(theta7)*sin(theta8)*sin(theta9) + 2*a2*mthigh*cos(theta3)*cos(theta4)*cos(theta5)*cos(theta6)*cos(theta8)*sin(theta7)*sin(theta9) + 2*a2*mthigh*cos(theta3)*cos(theta4)*cos(theta5)*cos(theta7)*cos(theta8)*sin(theta6)*sin(theta9) - lthigh*mthigh*cos(theta3)*cos(theta4)*cos(theta5)*cos(theta6)*cos(theta7)*sin(theta8)*sin(theta9) - lthigh*mthigh*cos(theta3)*cos(theta4)*cos(theta5)*cos(theta6)*cos(theta8)*sin(theta7)*sin(theta9) - lthigh*mthigh*cos(theta3)*cos(theta4)*cos(theta5)*cos(theta7)*cos(theta8)*sin(theta6)*sin(theta9) - 2*a2*mshank*cos(theta3)*cos(theta4)*cos(theta5)*sin(theta6)*sin(theta7)*sin(theta8)*sin(theta9) + 2*a2*mshank*cos(theta3)*cos(theta6)*cos(theta7)*sin(theta4)*sin(theta5)*sin(theta8)*sin(theta9) + 2*a2*mshank*cos(theta3)*cos(theta6)*cos(theta8)*sin(theta4)*sin(theta5)*sin(theta7)*sin(theta9) + 2*a2*mshank*cos(theta3)*cos(theta7)*cos(theta8)*sin(theta4)*sin(theta5)*sin(theta6)*sin(theta9) - 2*a2*mthigh*cos(theta3)*cos(theta4)*cos(theta5)*sin(theta6)*sin(theta7)*sin(theta8)*sin(theta9) + 2*a2*mthigh*cos(theta3)*cos(theta6)*cos(theta7)*sin(theta4)*sin(theta5)*sin(theta8)*sin(theta9) + 2*a2*mthigh*cos(theta3)*cos(theta6)*cos(theta8)*sin(theta4)*sin(theta5)*sin(theta7)*sin(theta9) + 2*a2*mthigh*cos(theta3)*cos(theta7)*cos(theta8)*sin(theta4)*sin(theta5)*sin(theta6)*sin(theta9) + lthigh*mthigh*cos(theta3)*cos(theta4)*cos(theta5)*sin(theta6)*sin(theta7)*sin(theta8)*sin(theta9) - lthigh*mthigh*cos(theta3)*cos(theta6)*cos(theta7)*sin(theta4)*sin(theta5)*sin(theta8)*sin(theta9) - lthigh*mthigh*cos(theta3)*cos(theta6)*cos(theta8)*sin(theta4)*sin(theta5)*sin(theta7)*sin(theta9) - lthigh*mthigh*cos(theta3)*cos(theta7)*cos(theta8)*sin(theta4)*sin(theta5)*sin(theta6)*sin(theta9) - 2*a2*mshank*cos(theta3)*sin(theta4)*sin(theta5)*sin(theta6)*sin(theta7)*sin(theta8)*sin(theta9) - 2*a2*mthigh*cos(theta3)*sin(theta4)*sin(theta5)*sin(theta6)*sin(theta7)*sin(theta8)*sin(theta9) + lthigh*mthigh*cos(theta3)*sin(theta4)*sin(theta5)*sin(theta6)*sin(theta7)*sin(theta8)*sin(theta9) + 2*a1*mshank*cos(theta2)*cos(theta3)*cos(theta4)*cos(theta5)*cos(theta6)*cos(theta7)*sin(theta8)*sin(theta9) + 2*a1*mshank*cos(theta2)*cos(theta3)*cos(theta4)*cos(theta5)*cos(theta6)*cos(theta8)*sin(theta7)*sin(theta9) + 2*a1*mshank*cos(theta2)*cos(theta3)*cos(theta4)*cos(theta5)*cos(theta7)*cos(theta8)*sin(theta6)*sin(theta9) - lshank*mshank*cos(theta2)*cos(theta3)*cos(theta4)*cos(theta5)*cos(theta6)*cos(theta7)*sin(theta8)*sin(theta9) - lshank*mshank*cos(theta2)*cos(theta3)*cos(theta4)*cos(theta5)*cos(theta6)*cos(theta8)*sin(theta7)*sin(theta9) - lshank*mshank*cos(theta2)*cos(theta3)*cos(theta4)*cos(theta5)*cos(theta7)*cos(theta8)*sin(theta6)*sin(theta9) - 2*a1*mshank*cos(theta2)*cos(theta3)*cos(theta4)*cos(theta5)*sin(theta6)*sin(theta7)*sin(theta8)*sin(theta9) + 2*a1*mshank*cos(theta2)*cos(theta3)*cos(theta6)*cos(theta7)*sin(theta4)*sin(theta5)*sin(theta8)*sin(theta9) + 2*a1*mshank*cos(theta2)*cos(theta3)*cos(theta6)*cos(theta8)*sin(theta4)*sin(theta5)*sin(theta7)*sin(theta9) + 2*a1*mshank*cos(theta2)*cos(theta3)*cos(theta7)*cos(theta8)*sin(theta4)*sin(theta5)*sin(theta6)*sin(theta9) - 2*a1*mshank*cos(theta4)*cos(theta5)*cos(theta6)*cos(theta7)*sin(theta2)*sin(theta3)*sin(theta8)*sin(theta9) - 2*a1*mshank*cos(theta4)*cos(theta5)*cos(theta6)*cos(theta8)*sin(theta2)*sin(theta3)*sin(theta7)*sin(theta9) - 2*a1*mshank*cos(theta4)*cos(theta5)*cos(theta7)*cos(theta8)*sin(theta2)*sin(theta3)*sin(theta6)*sin(theta9) + lshank*mshank*cos(theta2)*cos(theta3)*cos(theta4)*cos(theta5)*sin(theta6)*sin(theta7)*sin(theta8)*sin(theta9) - lshank*mshank*cos(theta2)*cos(theta3)*cos(theta6)*cos(theta7)*sin(theta4)*sin(theta5)*sin(theta8)*sin(theta9) - lshank*mshank*cos(theta2)*cos(theta3)*cos(theta6)*cos(theta8)*sin(theta4)*sin(theta5)*sin(theta7)*sin(theta9) - lshank*mshank*cos(theta2)*cos(theta3)*cos(theta7)*cos(theta8)*sin(theta4)*sin(theta5)*sin(theta6)*sin(theta9) + lshank*mshank*cos(theta4)*cos(theta5)*cos(theta6)*cos(theta7)*sin(theta2)*sin(theta3)*sin(theta8)*sin(theta9) + lshank*mshank*cos(theta4)*cos(theta5)*cos(theta6)*cos(theta8)*sin(theta2)*sin(theta3)*sin(theta7)*sin(theta9) + lshank*mshank*cos(theta4)*cos(theta5)*cos(theta7)*cos(theta8)*sin(theta2)*sin(theta3)*sin(theta6)*sin(theta9) - 2*a1*mshank*cos(theta2)*cos(theta3)*sin(theta4)*sin(theta5)*sin(theta6)*sin(theta7)*sin(theta8)*sin(theta9) + 2*a1*mshank*cos(theta4)*cos(theta5)*sin(theta2)*sin(theta3)*sin(theta6)*sin(theta7)*sin(theta8)*sin(theta9) - 2*a1*mshank*cos(theta6)*cos(theta7)*sin(theta2)*sin(theta3)*sin(theta4)*sin(theta5)*sin(theta8)*sin(theta9) - 2*a1*mshank*cos(theta6)*cos(theta8)*sin(theta2)*sin(theta3)*sin(theta4)*sin(theta5)*sin(theta7)*sin(theta9) - 2*a1*mshank*cos(theta7)*cos(theta8)*sin(theta2)*sin(theta3)*sin(theta4)*sin(theta5)*sin(theta6)*sin(theta9) + lshank*mshank*cos(theta2)*cos(theta3)*sin(theta4)*sin(theta5)*sin(theta6)*sin(theta7)*sin(theta8)*sin(theta9) - lshank*mshank*cos(theta4)*cos(theta5)*sin(theta2)*sin(theta3)*sin(theta6)*sin(theta7)*sin(theta8)*sin(theta9) + lshank*mshank*cos(theta6)*cos(theta7)*sin(theta2)*sin(theta3)*sin(theta4)*sin(theta5)*sin(theta8)*sin(theta9) + lshank*mshank*cos(theta6)*cos(theta8)*sin(theta2)*sin(theta3)*sin(theta4)*sin(theta5)*sin(theta7)*sin(theta9) + lshank*mshank*cos(theta7)*cos(theta8)*sin(theta2)*sin(theta3)*sin(theta4)*sin(theta5)*sin(theta6)*sin(theta9) + 2*a1*mshank*sin(theta2)*sin(theta3)*sin(theta4)*sin(theta5)*sin(theta6)*sin(theta7)*sin(theta8)*sin(theta9) - lshank*mshank*sin(theta2)*sin(theta3)*sin(theta4)*sin(theta5)*sin(theta6)*sin(theta7)*sin(theta8)*sin(theta9))/(4*mshank + 4*mthigh + 2*mtrunk);



VWcom=V_CoM;
AWcom=A_CoM;
